simulink library "SLUGS_Library"  (Simulink 7.8)
settings: Solver=ode45  SolverMode=SingleTasking  StartTime=0.0  StopTime=10.0  RelTol=1e-3
values from neighbouring files (symbols this model uses):
  apSampleTime = 0.01    [mcuInit.m]
  derivativesConstant = 5    [mcuInit.m]
  latlong_WP = 1    [mcuInit.m]
  T = 0.01    [mcuInit.m]
  Xpoints = [0 0]    [mcuInit.m]
  Ypoints = [0 0]    [mcuInit.m]
  Zpoints = [0 0]    [mcuInit.m]
undefined symbols (not defined in the file or in its folder): bankCommandLimit, barAdjust, baroCutTemp, baroOffset, baroScale, barTGain1, barTGain2, barTMean1, barTMean2, baseHeight, baseTemp, daLimit, deLimit, DiscIntNeverNeededParam, drLimit, dtLimit, gaind, getGSLocation, getWP, GS_location, Init_onlyOnce, Init_Reset, IPStar, ISA_g, lapseRate, mass, maxAcc, MaxDwnPthStar, maxDynPressure, maxEta, Ndelay, param, pitAdjust, pitchCommandLimit, pitCutTemp, pitotOffset, pitotScale, pitTGain1, pitTGain2, pitTMean1, pitTMean2, polesd, pressureSensorCutoff, rollControlLimit, SampleT, setDiagnosticFloat, setDiagnosticShort, setLogFloat1, setLogFloat2, setNavLong, setNavNav, tanIntercept, Ts, u1, y1, yawDamperLimit, yo, zerosd
libraries: SLUGS_Library x90, simulink x37, dsPICdrivers x33, aerolibconvert2 x4, aerolibutil x1, aerolibobsolete x1
(part 7 of 7)

== matlab function Navigation/Navigation/RTB/Follow Mobile Navigation/Zero out Z1 ==
  data: P output double; Pin input double
function P = P2D(Pin)
% This block supports an embeddable subset of the MATLAB language.
% See the help menu for details. 

P = [Pin(1); Pin(2); 0];

== matlab function Sensor Blocks/Pitot Sensor End/Tustin Lowpass, Auto Initial Condition3/Embedded MATLAB Function ==
  data: u input double; y output double; T input double; f input double
function y = fcn(u,T,f)
% This block supports an embeddable subset of the MATLAB language.
% See the help menu for details. 

persistent a
persistent b
persistent y_km1
persistent u_km1
if isempty(a)
    %tf = [T*omega/(2+T*omega) T*omega/(2+T*omega)],[1 (T*omega-2)/(T*omega+2)]
    %tf = [a a],[1 -b]
    omega = 2*pi*f;
    a=T*omega/(2+T*omega);
    b=-(T*omega-2)/(T*omega+2);
    y_km1=u;
    u_km1=u;
end

y = a*(u+u_km1)+b*y_km1;
y_km1=y;
u_km1=u;

== matlab function Navigation/Navigation/Zero out Z1 ==
  data: P output double; Pin input double
function P = P2D(Pin)
% This block supports an embeddable subset of the MATLAB language.
% See the help menu for details. 

P = [Pin(1); Pin(2); 0];

== matlab function Navigation/Navigation/Zero out Z2 ==
  data: P output double; Pin input double
function P = P2D(Pin)
% This block supports an embeddable subset of the MATLAB language.
% See the help menu for details. 

P = [Pin(1); Pin(2); 0];

== matlab function Navigation/Navigation/myMux Fun2 ==
  data: u1 input double; y output double; u2 input double; u3 input double
function y = myMux(u1, u2, u3)
% This block supports an embeddable subset of the MATLAB language.
% See the help menu for details. 

y = [u1(1); u2(1); u3(1)];

== matlab function Navigation/Navigation/myMux Fun5 ==
  data: u1 input double; y output double; u2 input double; u3 input double
function y = myMux(u1, u2, u3)
% This block supports an embeddable subset of the MATLAB language.
% See the help menu for details. 

y = [u1(1); u2(1); u3(1)];

== matlab function Navigation/Navigation/myMux Fun4 ==
  data: u1 input double; y output double; u2 input double; u3 input double
function y = myMux(u1, u2, u3)
% This block supports an embeddable subset of the MATLAB language.
% See the help menu for details. 

y = [u1(1); u2(1); u3(1)];

== matlab function Navigation/Navigation/myMux Fun3 ==
  data: u1 input double; y output double; u2 input double
function y = myMux(u1, u2)
% This block supports an embeddable subset of the MATLAB language.
% See the help menu for details. 

y = [u1(1); u1(2); u2(1)];

== matlab function Navigation/Navigation/Circle Navigation/Get SP Location/Zero out Z2 ==
  data: P output double; Pin input double
function P = P2D(Pin)
% This block supports an embeddable subset of the MATLAB language.
% See the help menu for details. 

P = [Pin(1); Pin(2); 0];

== matlab function Navigation/Navigation/Circle Navigation/Inside the Circle, Keep Straight until intersection/Compute Head of Circle ==
  data: R input double; topCoord output double; ISR input double
function topCoord = getLocation(R, ISR)
%% Compute the top coordinate of the circle
% using the circle's parametric equations:
%  x = a + r cos (t)
%  y = b + r sin (t)
%
% @ t =0

topCoord = zeros(3,1);

topCoord(1) = ISR(1)+ R;
topCoord(2) = ISR(2);
topCoord(3) = ISR(3);

== matlab function Navigation/Navigation/myMux Fun1 ==
  data: u1 input double; y output double; u2 input double; u3 input double; u4 input double
function y = FeedNavNavAcordingToMode(u1, u2, u3, u4)
% This block supports an embeddable subset of the MATLAB language.
% See the help menu for details. 
y = [u1(1); u2(1); u3(1); u4(1)];

== matlab function Compute Angle Between Vectors/negprotect3 ==
  data: val input double; zpVal output double
function zpVal = negProt(val)
% This block supports an embeddable subset of the MATLAB language.
% See the help menu for details. 

if val >= single(0.0001)
    zpVal = val;
else
    zpVal = single(0.0001);
end

== matlab function Navigation/Navigation/Circle Navigation/Intersection. Circular Navigation/Embedded MATLAB Function ==
  data: hFact input double; P31 output double; P2 input double; P32 output double
function [P31,P32] = getP3s(hFact, P2)
% This block supports an embeddable subset of the MATLAB language.
% See the help menu for details. 

P31 = single([0 0 0]');
P32 = single([0 0 0]');

P31(1) = P2(1) + hFact(2);
P32(1) = P2(1) - hFact(2);

P31(2) = P2(2) - hFact(1);
P32(2) = P2(2) + hFact(1);

== matlab function Navigation/Navigation/Circle Navigation/Intersection. Circular Navigation/negprotect1 ==
  data: val input double; zpVal output double
function zpVal = negProt(val)
% This block supports an embeddable subset of the MATLAB language.
% See the help menu for details. 

if val >= single(0.0001)
    zpVal = val;
else
    zpVal = single(0.0001);
end

== matlab function Navigation/Navigation/Circle Navigation/Intersection. Circular Navigation/negprotect2 ==
  data: val input double; zpVal output double
function zpVal = negProt(val)
% This block supports an embeddable subset of the MATLAB language.
% See the help menu for details. 

if val >= single(0.0001)
    zpVal = val;
else
    zpVal = single(0.0001);
end
